simulink model "a1_waypoint"  (R2021b)
settings: Solver=FixedStepAuto  StartTime=0.0  StopTime=30  FixedStep=0.1  RelTol=1e-3
PreLoadFcn:
  | % Simulation parameters
  | %load exampleMap
InitFcn:
  | sampleTime = 0.05;
  | 
  | % Robot parameters
  | wheelRadius = 0.025;
  | robotRadius = 0.15;
  | 
  | % Lidar parameters
  | sensorOffset = [0,0];
  | scanAngles = linspace(-pi/2,pi/2,9)';
  | maxRange = 5;
  | 
  | %%%%%%
  | ks=1;
  | 
  | %初始位置
  | x_1_0=0;
  | y_1_0=0;
  | yaw_1_0=0;
  | 
  | x_2_0=0;
  | y_2_0=0.3;
  | yaw_2_0=0;
  | 
  | x_3_0=0;
  | y_3_0=0.6;
  | yaw_3_0=0;
  | 
  | x_4_0=0;
  | y_4_0=0.9;
  | yaw_4_0=0;
  | 
  | 
  | A=0.3;
  | C=1.7;
  | B=(A+C)/2;
  | 
  | wp1=[A,A; B,A;  C,A; C,B;C,C; B,C; A,C;A,B];
  | WAY_P=[wp1;wp1;wp1;wp1];
libraries: mobileRoboticsLib x1, robotmobilelib x1
settings Model: SimulationMode=accelerator  Creator=scastro  LastModifiedBy=amov
settings SolverCC: AlgebraicLoopSolver=TrustRegion
settings DataIOCC: ReturnWorkspaceOutputs=off
settings OptimizationCC: EnhancedBackFolding=on  PassReuseOutputArgsAs=Individual arguments  ZeroExternalMemoryAtStartup=off  ZeroInternalMemoryAtStartup=off  MaxStackSize=64  OptimizeBlockOrder=speed  DifferentSizesBufferReuse=on  OptimizationCustomize=off  EfficientTunableParamExpr=on
settings DebuggingCC: ParameterTunabilityLossMsg=error  PregeneratedLibrarySubsystemCodeDiagnostic=none  SFMachineParentedDataDiag=warning  ArithmeticOperatorsInVariantConditions=warning
settings HardwareCC: ProdBitPerPointer=32  ProdBitPerSizeT=32  ProdBitPerPtrDiffT=32  ProdLargestAtomicFloat=None  ProdIntDivRoundTo=Undefined  ProdEndianess=Unspecified  ProdWordSize=32  ProdHWDeviceType=Generic->Unspecified (assume 32-bit Generic)
settings SFSimCC: SimUseLocalCustomCode=off  MATLABDynamicMemAlloc=off  CustomCodeUndefinedFunction=UseInterfaceOnly
settings RTWCC: Description=Embedded Coder  SystemTargetFile=ert.tlc  HardwareBoard=Robot Operating System (ROS)  TLCOptions="-aInlineSetEventsForThisBaseRateFcn=TLC_FALSE -aSuppressMultiTaskScheduler=TLC_FALSE  -aRateBasedStepFcn=0"  TemplateMakefile=ert_default_tmf  RTWUseLocalCustomCode=off  Toolchain=Catkin  TargetLang=C++
settings CodeAppCC: ForceParamTrailComments=on  IgnoreCustomStorageClasses=off  OperatorAnnotations=on  SimulinkDataObjDesc=on  SFDataObjDesc=on  InsertBlockDesc=on

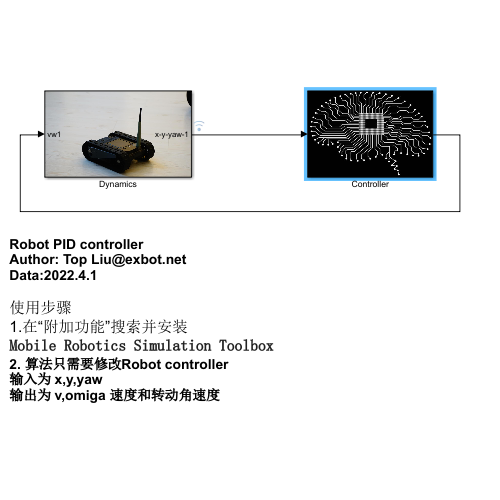
[thumbnail: Simulink's stored preview of the top-level diagram]
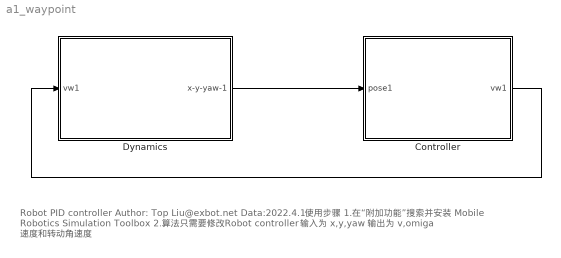
== system a1_waypoint ==
  note: Robot PID controller
      | Author: Top Liu@exbot.net
      | Data:2022.4.1
      |
      | 使用步骤
      | 1.在“附加功能”搜索并安装
      | Mobile Robotics Simulation Toolbox
      | 2. 算法只需要修改Robot controller
      | 输入为 x,y,yaw
      | 输出为 v,omiga 速度和转动角速度
  Controller : Subsystem
      mask Display: image('$imagefile'); % 使用工具条上的 "编辑图像" 进行更改。
  Dynamics : Subsystem
      mask Display: image('$imagefile'); % 使用工具条上的 "编辑图像" 进行更改。
  wires:
  Controller/1(vw1) -> Dynamics/1(vw1)
  Dynamics/1(x-y-yaw-1) -> Controller/1(pose1)

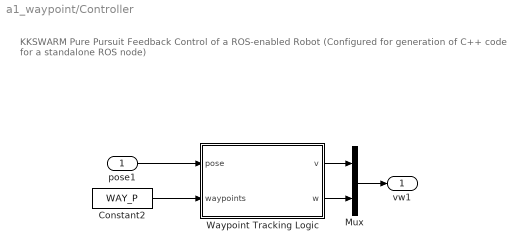
== system a1_waypoint/Controller ==
  note: KKSWARM Pure Pursuit Feedback Control of a ROS-enabled Robot
      | (Configured for generation of C++ code for a standalone ROS node)
  pose1 : Inport
  Constant2 : Constant  Value=WAY_P
  Mux : Mux  Inputs=2
  Waypoint Tracking Logic : Stateflow chart  TreatAsAtomicUnit=on
  vw1 : Outport
  wires:
  Waypoint Tracking Logic/1(v) -> Mux/1
  pose1/1 -> Waypoint Tracking Logic/1(pose)
  Mux/1 -> vw1/1
  Waypoint Tracking Logic/2(w) -> Mux/2
  Constant2/1 -> Waypoint Tracking Logic/2(waypoints)

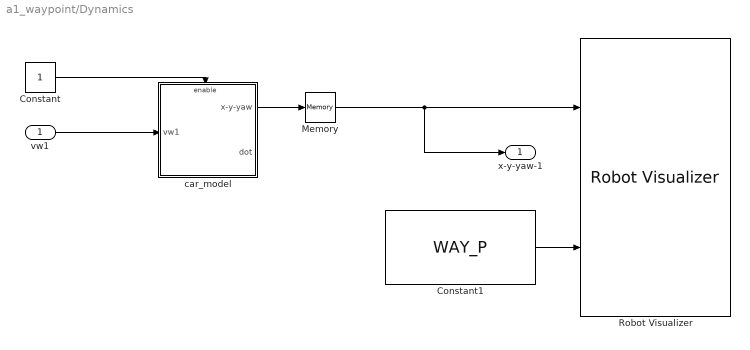
== system a1_waypoint/Dynamics ==
  vw1 : Inport
  Constant : Constant
  Constant1 : Constant  Value=WAY_P
  Memory : Memory  InheritSampleTime=on
  Robot Visualizer : mobileRoboticsLib/Environments/Robot Visualizer  Priority=99  robotRadius=0.15  showTrajectory=on  hasWaypoints=on  hasLidar=off  sensorOffset=scanSensorOffset  scanAngles=scanAngles  hasObjDetector=off  objDetectorOffset=[ 0, 0 ]  objDetectorAngle=0  objDetectorFOV=0  objDetectorMaxRange=0  objectColors=0  objectMarkers='s'
  car_model : Subsystem
  x-y-yaw-1 : Outport
  wires:
  Constant/1 -> car_model/Enable
  Memory/1 -> x-y-yaw-1/1, Robot Visualizer/1
  vw1/1 -> car_model/1(vw1)
  Constant1/1 -> Robot Visualizer/2
  car_model/1(x-y-yaw) -> Memory/1

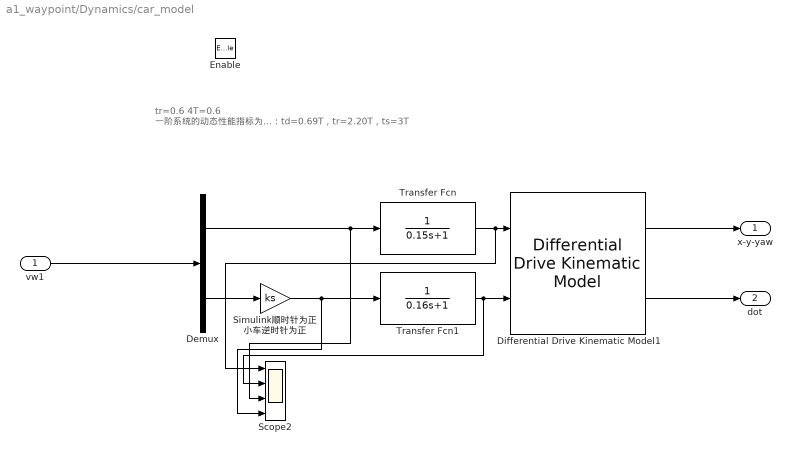
== system a1_waypoint/Dynamics/car_model ==
  note: tr=0.6
      | 4T=0.6
      | 一阶系统的动态性能指标为：td=0.69T，tr=2.20T，ts=3T
  vw1 : Inport
  Enable : EnablePort  ShowOutputPort=on
  Demux : Demux  Outputs=2
  Differential Drive Kinematic Model1 : robotmobilelib/Differential Drive Kinematic Model  VehicleInputs=Vehicle Speed & Heading Angular Velocity  WheelRadius=0.05  WheelSpeedRange=[-inf inf]  TrackWidth=0.2  InitialState=[x_1_0, y_1_0, yaw_1_0]'  SimulateUsing=Interpreted execution
      settings: SourceProductBaseCode=RO
  Scope2 : Scope  NumInputPorts=4
  Simulink顺时针为正 小车逆时针为正 : Gain  Gain=ks
  Transfer Fcn : TransferFcn  Denominator=[0.15 1]
  Transfer Fcn1 : TransferFcn  Denominator=[0.16 1]
  x-y-yaw : Outport
  dot : Outport  Port=2
  wires:
  Simulink顺时针为正 小车逆时针为正/1 -> Scope2/4, Transfer Fcn1/1
  Transfer Fcn/1 -> Differential Drive Kinematic Model1/1, Scope2/1
  Demux/1 -> Scope2/3, Transfer Fcn/1
  Transfer Fcn1/1 -> Differential Drive Kinematic Model1/2, Scope2/2
  Demux/2 -> Simulink顺时针为正 小车逆时针为正/1
  vw1/1 -> Demux/1
  Differential Drive Kinematic Model1/1 -> x-y-yaw/1
  Differential Drive Kinematic Model1/2 -> dot/1

== stateflow chart a1_waypoint/Controller/Waypoint Tracking Logic ==
  state FollowWaypoints
    entry:
    goalPoint = waypoints(idx,:);
    entry, during:
    [angle,range] = trackGoal(goalPoint);
    (default) -> (junction 20)
    FollowWaypoints -> (junction 20) [order 1]
    (junction 20) -> (junction 24) [order 1] : % Set angular speed if
        | % angle outside deadband
        | [abs(angle) > pi/24]
    (junction 20) -> (junction 30) [order 2] : {w = 0;}
    (junction 24) -> (junction 49) : % Proportional
        | % control
        | {w = 1.5*angle;}
    (junction 49) -> (junction 30)
  state ReachedGoal
    entry:
    v = 0;
    w = 0.5;
  (default) -> FollowWaypoints : {
      | v = 0.3;
      | idx = 1;
      | numPts = size(waypoints,1);
      | }
  FollowWaypoints -> (junction 39) [order 1] : % Check if goal reached
      | [range < 0.2]
  (junction 39) -> ReachedGoal [order 1] : % Stop if final waypoint
      | [idx == numPts]
  (junction 39) -> (junction 42) [order 2]
  (junction 42) -> FollowWaypoints : % Go to the next waypoint
      | {idx = idx + 1;}
  data: goal function_input; ang function_output; dist function_output; pose input; waypoints input; v output; w output; angle local; range local; idx local; numPts local; goalPoint local
  function [ang,dist] = trackGoal(goal):
    | function [ang,dist] = trackGoal(goal)
    | % Finds the angle (theta) and distance (dist) between the 
    | % vehicle and a goal point
    |     
    | posDiff = [goal(1)-pose(1);goal(2)-pose(2)];
    | 
    | ang = angdiff(pose(3),atan2(posDiff(2),posDiff(1)));
    | dist = sqrt(posDiff(1)^2 + posDiff(2)^2);
